simulink model "testichannel"  (Simulink 7.1)
settings: Solver=ode45  StartTime=0.0  StopTime=0.0  RelTol=1e-3
undefined symbols (not defined in the file): IScale
libraries: SaliencyLib x1
settings Model: Creator=bruce  LastModifiedBy=bruce

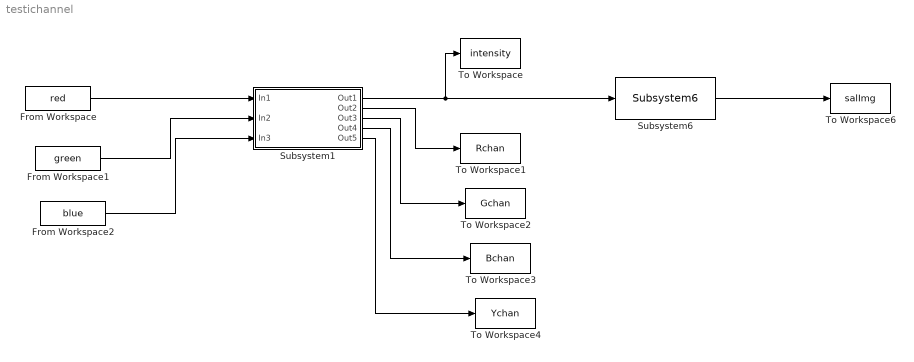
== system testichannel ==
  From Workspace : FromWorkspace  VariableName=red  SampleTime=0
  From Workspace1 : FromWorkspace  VariableName=green  SampleTime=0
  From Workspace2 : FromWorkspace  VariableName=blue  SampleTime=0
  Subsystem1 : Subsystem
      mask Display:
      | disp('COLOR\nMAPPING')
      | port_label('input',1,'r')
      | port_label('input',2','g')
      | port_label('input',3,'b')
      | port_label('output',1,'I')
      | port_label('output',2,'R')
      | port_label('output',3,'G')
      | port_label('output',4','B')
      | port_label('output',5,'Y')
  Subsystem6 : SaliencyLib/Subsystem6  SystemSampleTime=-1  isr=332  isc=500
      link override Subsystem17/Level-2 M-file S-Function: br=83  bc=125
      link override Subsystem17/Level-2 M-file S-Function1: sr=83  sc=125
      link override Subsystem17/Level-2 M-file S-Function2: sr=83  sc=125
      link override Subsystem17/Level-2 M-file S-Function3: sr=42  sc=63
      link override Subsystem17/Level-2 M-file S-Function4: sr=42  sc=63
      link override Subsystem17/Level-2 M-file S-Function5: br=83  bc=125
      link override Subsystem17/Level-2 M-file S-Function6: br=42  bc=63
      link override Subsystem17/Level-2 M-file S-Function7: br=42  bc=63
  To Workspace : ToWorkspace  VariableName=intensity  SampleTime=-1  SaveFormat=Structure
  To Workspace1 : ToWorkspace  VariableName=Rchan  SampleTime=-1  SaveFormat=Structure
  To Workspace2 : ToWorkspace  VariableName=Gchan  SampleTime=-1  SaveFormat=Structure
  To Workspace3 : ToWorkspace  VariableName=Bchan  SampleTime=-1  SaveFormat=Structure
  To Workspace4 : ToWorkspace  VariableName=Ychan  SampleTime=-1  SaveFormat=Structure
  To Workspace6 : ToWorkspace  VariableName=salImg  SampleTime=-1  SaveFormat=Structure
  wires:
  From Workspace/1 -> Subsystem1/1(In1)
  Subsystem1/1(Out1) -> To Workspace/1, Subsystem6/1
  From Workspace1/1 -> Subsystem1/2(In2)
  From Workspace2/1 -> Subsystem1/3(In3)
  Subsystem1/2(Out2) -> To Workspace1/1
  Subsystem1/3(Out3) -> To Workspace2/1
  Subsystem1/4(Out4) -> To Workspace3/1
  Subsystem1/5(Out5) -> To Workspace4/1
  Subsystem6/1 -> To Workspace6/1

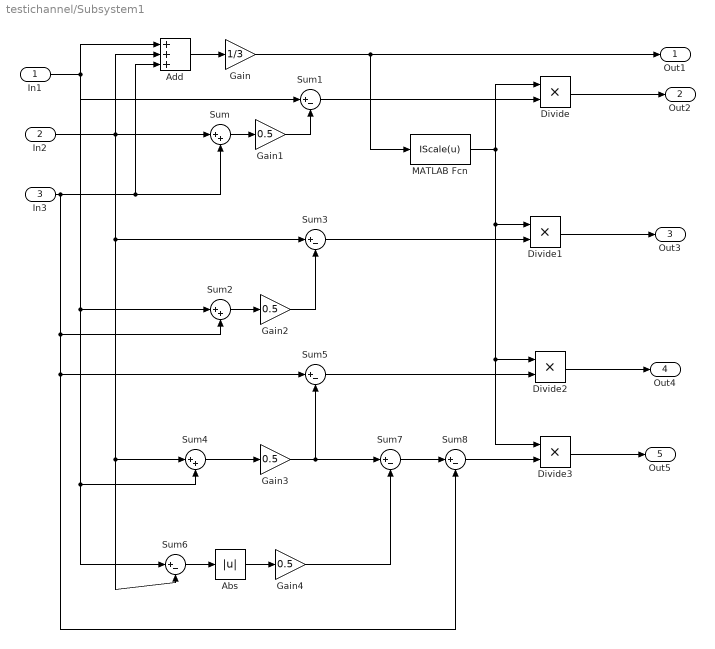
== system testichannel/Subsystem1 ==
  In1 : Inport  OutDataType=sfix(16)  OutScaling=2^0
  In2 : Inport  Port=2  OutDataType=sfix(16)  OutScaling=2^0
  In3 : Inport  Port=3  OutDataType=sfix(16)  OutScaling=2^0
  Abs : Abs  OutDataType=sfix(16)  OutScaling=2^0
  Add : Sum  Inputs=+++  OutDataType=sfix(16)  OutScaling=2^-10
  Divide{,1..3} (4 alike) : Product  Inputs=**  OutDataType=sfix(16)  OutScaling=2^-10
  Gain : Gain  Gain=1/3  ParameterDataType=sfix(16)  ParameterScaling=2^0  OutDataType=sfix(16)  OutScaling=2^0
  Gain{1..4} (4 alike) : Gain  Gain=0.5  ParameterDataType=sfix(16)  ParameterScaling=2^0  OutDataType=sfix(16)  OutScaling=2^0
  MATLAB Fcn : MATLABFcn  MATLABFcn=IScale(u)  Output1D=off
  Sum : Sum  Inputs=|++  OutDataType=sfix(16)  OutScaling=2^0
  Sum{1,3,5..8} (6 alike) : Sum  Inputs=|+-  OutDataType=sfix(16)  OutScaling=2^0
  Sum2 : Sum  Inputs=|++  OutDataType=sfix(16)  OutScaling=2^0
  Sum4 : Sum  Inputs=|++  OutDataType=sfix(16)  OutScaling=2^0
  Out1 : Outport  OutDataType=sfix(16)  OutScaling=2^0
  Out2 : Outport  Port=2  OutDataType=sfix(16)  OutScaling=2^0
  Out3 : Outport  Port=3  OutDataType=sfix(16)  OutScaling=2^0
  Out4 : Outport  Port=4  OutDataType=sfix(16)  OutScaling=2^0
  Out5 : Outport  Port=5  OutDataType=sfix(16)  OutScaling=2^0
  wires:
  MATLAB Fcn/1 -> Divide3/1, Divide2/1, Divide1/1, Divide/1
  Divide3/1 -> Out5/1
  Sum8/1 -> Divide3/2
  Sum7/1 -> Sum8/1
  Gain4/1 -> Sum7/2
  Abs/1 -> Gain4/1
  Sum6/1 -> Abs/1
  Divide2/1 -> Out4/1
  Divide1/1 -> Out3/1
  Sum5/1 -> Divide2/2
  Sum3/1 -> Divide1/2
  Divide/1 -> Out2/1
  Sum1/1 -> Divide/2
  Sum4/1 -> Gain3/1
  Gain3/1 -> Sum7/1, Sum5/2
  Gain2/1 -> Sum3/2
  Sum2/1 -> Gain2/1
  Gain1/1 -> Sum1/2
  Sum/1 -> Gain1/1
  Add/1 -> Gain/1
  Gain/1 -> MATLAB Fcn/1, Out1/1
  In3/1 -> Sum8/2, Sum5/1, Sum2/2, Sum/2, Add/3
  In2/1 -> Sum6/2, Sum4/1, Sum3/1, Sum/1, Add/2
  In1/1 -> Sum6/1, Sum4/2, Sum2/1, Sum1/1, Add/1
